simulink model "ENBW_test_simulink"  (R2021a)
settings: Solver=ode4  StartTime=0.0  StopTime=50.0  FixedStep=0.001  RelTol=1e-3
settings Model: Creator=longt  LastModifiedBy=longt
settings DataIOCC: SaveOutput=off  SignalLogging=off  DSMLogging=off  SaveTime=off  ReturnWorkspaceOutputs=off

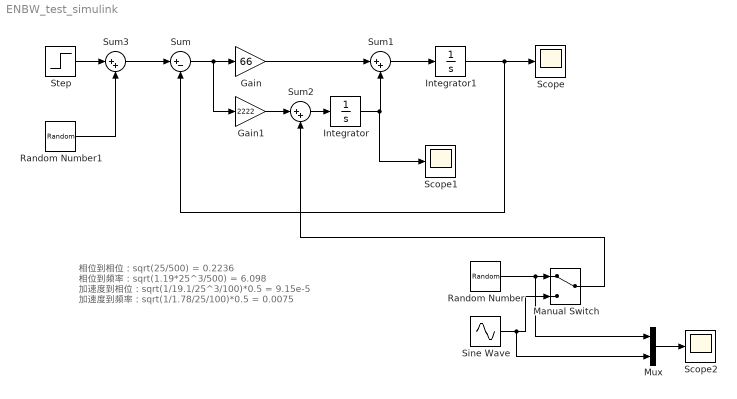
== system ENBW_test_simulink ==
  note: 相位到相位：sqrt(25/500) = 0.2236
      | 相位到频率：sqrt(1.19*25^3/500) = 6.098
      | 加速度到相位：sqrt(1/19.1/25^3/100)*0.5 = 9.15e-5
      | 加速度到频率：sqrt(1/1.78/25/100)*0.5 = 0.0075
  Gain : Gain  Gain=66
  Gain1 : Gain  Gain=2222
  Integrator : Integrator
  Integrator1 : Integrator
  Manual Switch : ManualSwitch
  Mux : Mux  Inputs=2
  Random Number : RandomNumber  Variance=(0.1*5)^2*1  SampleTime=0.01
  Random Number1 : RandomNumber  Variance=1^2*0  SampleTime=0.001
  Scope : Scope
  Scope1 : Scope
  Scope2 : Scope
  Sine Wave : Sin  Amplitude=0.5  Frequency=20*2*pi  SampleTime=0.01
  Step : Step  Time=100  SampleTime=0
  Sum : Sum  Inputs=|+-
  Sum1 : Sum  Inputs=|++
  Sum2 : Sum  Inputs=|++
  Sum3 : Sum  Inputs=|++
  wires:
  Sum/1 -> Gain1/1, Gain/1
  Gain/1 -> Sum1/1
  Integrator/1 -> Scope1/1, Sum1/2
  Sum1/1 -> Integrator1/1
  Integrator1/1 -> Sum/2, Scope/1
  Gain1/1 -> Sum2/1
  Sum2/1 -> Integrator/1
  Step/1 -> Sum3/1
  Sum3/1 -> Sum/1
  Random Number1/1 -> Sum3/2
  Random Number/1 -> Mux/1, Manual Switch/1
  Sine Wave/1 -> Mux/2, Manual Switch/2
  Manual Switch/1 -> Sum2/2
  Mux/1 -> Scope2/1
